simulink model "CompleteModel"  (R2020b)
settings: Solver=ode23t  StartTime=0.0  StopTime=6000  RelTol=1e-3
values from neighbouring files (symbols this model uses):
  alpha_1 = 0.5019    [Data_Parameters_CompleteModel.m]
  alpha_2 = 0.4982    [Data_Parameters_CompleteModel.m]
  Cp = 3200    [Data_Parameters_CompleteModel.m]
  D = [-D2 0 -D4 -2*D5 ... (first row only)    [Data_Parameters_CompleteModel.m]
  d = 1.5e-6    (= 1.5e-06)    [Data_Parameters_CompleteModel.m]
  D2 = 4.438e-14    [Data_Parameters_CompleteModel.m]
  D3 = 1.0024e-14    [Data_Parameters_CompleteModel.m]
  D4 = 3.8e-14    [Data_Parameters_CompleteModel.m]
  D5 = 1.75e-14    [Data_Parameters_CompleteModel.m]
  D_col = 2*A_col/(h_col+w_col)    (= 0.0193548387097)    [Data_Parameters_CompleteModel.m]
  D_L1 = [D_L11 D_L12 D_L13]    [Data_Parameters_CompleteModel.m]
  D_L2 = [D_L21 D_L22 D_L23]    [Data_Parameters_CompleteModel.m]
  D_rec = 2*A_rec/(w_rec+t_rec)    (= 0.00248962655602)    [Data_Parameters_CompleteModel.m]
  F = 96485    [Data_Parameters_CompleteModel.m]
  f_L1 = [f_L11 f_L12 f_L13]    [Data_Parameters_CompleteModel.m]
  f_L2 = [f_L21 f_L22 f_L23]    [Data_Parameters_CompleteModel.m]
  f_value = 58.91    [Data_Parameters_CompleteModel.m]
  H1 = -220000    [Data_Parameters_CompleteModel.m]
  H2 = -64000    [Data_Parameters_CompleteModel.m]
  H4 = -91200    [Data_Parameters_CompleteModel.m]
  H5 = -246800    [Data_Parameters_CompleteModel.m]
  h_col = 0.01    [Data_Parameters_CompleteModel.m]
  k0_1 = 1.6e-6    (= 1.6e-06)    [Data_Parameters_CompleteModel.m]
  k0_2 = 1.5e-4    (= 0.00015)    [Data_Parameters_CompleteModel.m]
  K_con1 = 0.35    [Data_Parameters_CompleteModel.m]
  K_con2 = 0.35    [Data_Parameters_CompleteModel.m]
  K_dec1 = 0.07    [Data_Parameters_CompleteModel.m]
  K_dec2 = 0.07    [Data_Parameters_CompleteModel.m]
  K_E1 = [K_E11 K_E12 K_E13]    [Data_Parameters_CompleteModel.m]
  K_E2 = [K_E21 K_E22 K_E23]    [Data_Parameters_CompleteModel.m]
  K_el = (df^2/(16*CKC))*(porosity^3/(1-porosity)^2)*w_el*t_el    (= 2.96777943925e-13)    [Data_Parameters_CompleteModel.m]
  K_exp1 = 0.7    [Data_Parameters_CompleteModel.m]
  K_exp2 = 0.7    [Data_Parameters_CompleteModel.m]
  K_in1 = 0.5    [Data_Parameters_CompleteModel.m]
  K_in2 = 0.5    [Data_Parameters_CompleteModel.m]
  K_inc1 = 0.68    [Data_Parameters_CompleteModel.m]
  K_inc2 = 0.68    [Data_Parameters_CompleteModel.m]
  K_out1 = 1.0    (= 1)    [Data_Parameters_CompleteModel.m]
  K_out2 = 1.0    (= 1)    [Data_Parameters_CompleteModel.m]
  K_valve1 = 0.06    [Data_Parameters_CompleteModel.m]
  K_valve2 = 0.06    [Data_Parameters_CompleteModel.m]
  Kin = 0.5    [Data_Parameters_CompleteModel.m]
  Kout = 1.0    (= 1)    [Data_Parameters_CompleteModel.m]
  L_col = 0.53    [Data_Parameters_CompleteModel.m]
  L_el = 0.3    [Data_Parameters_CompleteModel.m]
  L_L1 = [L_L11 L_L12 L_L13]    [Data_Parameters_CompleteModel.m]
  L_L2 = [L_L21 L_L22 L_L23]    [Data_Parameters_CompleteModel.m]
  L_rec = 0.02    [Data_Parameters_CompleteModel.m]
  mu = 4.928e-3    (= 0.004928)    [Data_Parameters_CompleteModel.m]
  N = 1    [Data_Parameters_CompleteModel.m]
  N_E1 = [N_E11 N_E12 N_E13]    [Data_Parameters_CompleteModel.m]
  N_E2 = [N_E21 N_E22 N_E23]    [Data_Parameters_CompleteModel.m]
  N_in1 = 2    [Data_Parameters_CompleteModel.m]
  N_in2 = 2    [Data_Parameters_CompleteModel.m]
  N_out1 = 2    [Data_Parameters_CompleteModel.m]
  N_out2 = 2    [Data_Parameters_CompleteModel.m]
  N_valves1 = 3    [Data_Parameters_CompleteModel.m]
  N_valves2 = 3    [Data_Parameters_CompleteModel.m]
  r = 0.04    [Data_Parameters_CompleteModel.m]
  R = 8.31    [Data_Parameters_CompleteModel.m]
  ro = 1354    [Data_Parameters_CompleteModel.m]
  S = 9e-4    (= 0.0009)    [Data_Parameters_CompleteModel.m]
  T = 298    [Data_Parameters_CompleteModel.m]
  t_rec = 0.00125    [Data_Parameters_CompleteModel.m]
  UpAp = 0.47    [Data_Parameters_CompleteModel.m]
  UsAs = 1.31    [Data_Parameters_CompleteModel.m]
  UtAt = 12.69    [Data_Parameters_CompleteModel.m]
  Vcell = 0.0171    [Data_Parameters_CompleteModel.m]
  Vpipe = 1.256e-3    (= 0.001256)    [Data_Parameters_CompleteModel.m]
  Vtank_Anolyte = 45e-6    (= 4.5e-05)    [Data_Parameters_CompleteModel.m]
  Vtank_Catholyte = 55.74e-6    (= 5.574e-05)    [Data_Parameters_CompleteModel.m]
  w_col = 0.3    [Data_Parameters_CompleteModel.m]
  w_rec = 0.3    [Data_Parameters_CompleteModel.m]
undefined symbols (not defined in the file or in its folder): magnitude
(part 2 of 2)

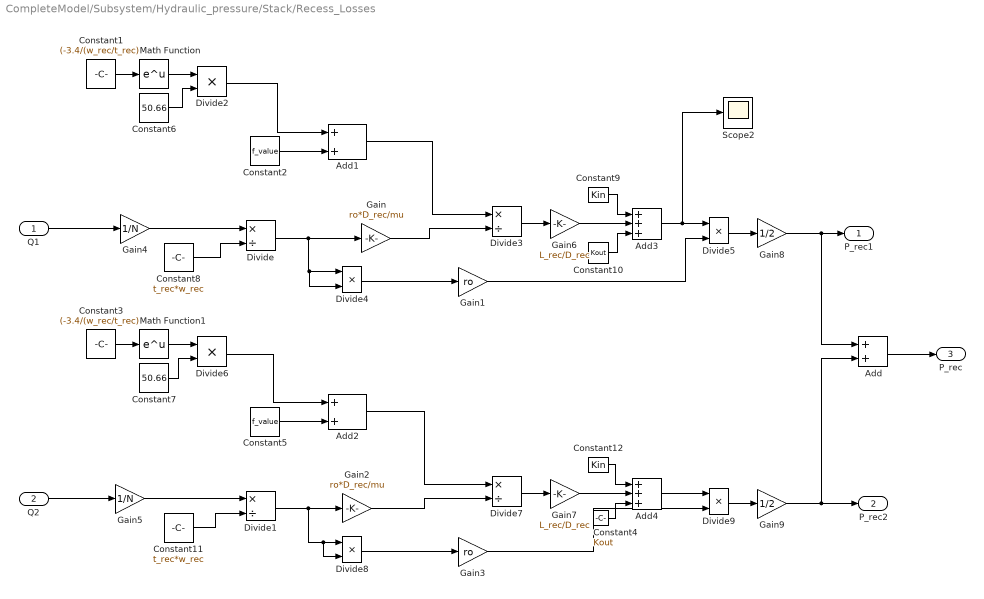
== system CompleteModel/Subsystem/Hydraulic_pressure/Stack/Recess_Losses ==
  Q1 : Inport
  Q2 : Inport  Port=2
  Add : Sum
  Add1 : Sum
  Add2 : Sum
  Add3 : Sum  Inputs=+++
  Add4 : Sum  Inputs=+++
  Constant1 : Constant  Value=(-3.4/(w_rec/t_rec))
  Constant10 : Constant  Value=Kout
  Constant11 : Constant  Value=t_rec*w_rec
  Constant12 : Constant  Value=Kin
  Constant2 : Constant  Value=f_value
  Constant3 : Constant  Value=(-3.4/(w_rec/t_rec))
  Constant4 : Constant  Value=Kout
  Constant5 : Constant  Value=f_value
  Constant6 : Constant  Value=50.66
  Constant7 : Constant  Value=50.66
  Constant8 : Constant  Value=t_rec*w_rec
  Constant9 : Constant  Value=Kin
  Divide{,1,3,7} (4 alike) : Product  Inputs=*/
  Divide{2,4..6,8..9} (6 alike) : Product  Inputs=**
  Gain : Gain  Gain=ro*D_rec/mu
  Gain1 : Gain  Gain=ro
  Gain2 : Gain  Gain=ro*D_rec/mu
  Gain3 : Gain  Gain=ro
  Gain4 : Gain  Gain=1/N
  Gain5 : Gain  Gain=1/N
  Gain6 : Gain  Gain=L_rec/D_rec
  Gain7 : Gain  Gain=L_rec/D_rec
  Gain8 : Gain  Gain=1/2
  Gain9 : Gain  Gain=1/2
  Math Function : Math  SignedPower=on  SaturateOnIntegerOverflow=on
  Math Function1 : Math  SignedPower=on  SaturateOnIntegerOverflow=on
  Scope2 : Scope
  P_rec1 : Outport  VectorParamsAs1DForOutWhenUnconnected=off
  P_rec2 : Outport  Port=2  VectorParamsAs1DForOutWhenUnconnected=off
  P_rec : Outport  Port=3  VectorParamsAs1DForOutWhenUnconnected=off
  wires:
  Q1/1 -> Gain4/1
  Constant8/1 -> Divide/2
  Divide/1 -> Divide4/2, Divide4/1, Gain/1
  Constant1/1 -> Math Function/1
  Math Function/1 -> Divide2/1
  Gain/1 -> Divide3/2
  Add1/1 -> Divide3/1
  Divide5/1 -> Gain8/1
  Add/1 -> P_rec/1
  Constant2/1 -> Add1/2
  Divide2/1 -> Add1/1
  Constant6/1 -> Divide2/2
  Divide4/1 -> Gain1/1
  Divide3/1 -> Gain6/1
  Constant10/1 -> Add3/3
  Constant9/1 -> Add3/1
  Add3/1 -> Scope2/1, Divide5/1
  Gain1/1 -> Divide5/2
  Divide8/1 -> Gain3/1
  Constant4/1 -> Add4/3
  Gain3/1 -> Divide9/2
  Constant12/1 -> Add4/1
  Add4/1 -> Divide9/1
  Constant3/1 -> Math Function1/1
  Constant7/1 -> Divide6/2
  Divide6/1 -> Add2/1
  Add2/1 -> Divide7/1
  Divide7/1 -> Gain7/1
  Constant5/1 -> Add2/2
  Divide1/1 -> Divide8/1, Divide8/2, Gain2/1
  Q2/1 -> Gain5/1
  Math Function1/1 -> Divide6/1
  Constant11/1 -> Divide1/2
  Gain2/1 -> Divide7/2
  Divide9/1 -> Gain9/1
  Gain4/1 -> Divide/1
  Gain5/1 -> Divide1/1
  Gain6/1 -> Add3/2
  Gain7/1 -> Add4/2
  Gain8/1 -> Add/1, P_rec1/1
  Gain9/1 -> P_rec2/1, Add/2
